simulink model "smart_irrigation_system_sim"  (R2021a)
settings: Solver=VariableStepAuto  StartTime=0.0  StopTime=10.0  RelTol=1e-3
libraries: spsBistableLib x1
settings Model: Creator=samad  LastModifiedBy=samad

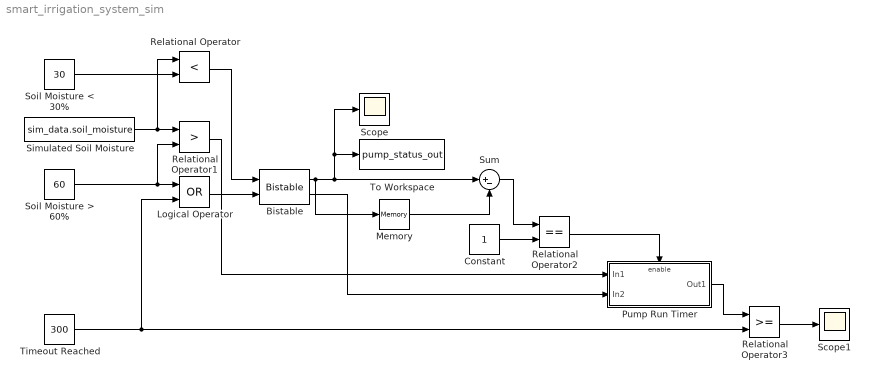
== system smart_irrigation_system_sim ==
  Bistable : spsBistableLib/Bistable  Qpriority=Set  ic=0  Ts=-1
      settings: SourceProductBaseCode=PS
  Constant : Constant
  Logical Operator : Logic  Operator=OR  AllPortsSameDT=off  OutDataTypeStr=boolean
  Memory : Memory
  Pump Run Timer : Subsystem  TreatAsAtomicUnit=on
  Relational Operator : RelationalOperator  Operator=<  OutDataTypeStr=boolean  RndMeth=Simplest
  Relational Operator1 : RelationalOperator  Operator=>  OutDataTypeStr=boolean  RndMeth=Simplest
  Relational Operator2 : RelationalOperator  Operator===  OutDataTypeStr=boolean  RndMeth=Simplest
  Relational Operator3 : RelationalOperator  OutDataTypeStr=boolean  RndMeth=Simplest
  Scope : Scope
  Scope1 : Scope
  Simulated Soil Moisture : FromWorkspace  VariableName=sim_data.soil_moisture  SampleTime=5/60
  Soil Moisture < 30% : Constant  Value=30
  Soil Moisture > 60% : Constant  Value=60
  Sum : Sum  Inputs=|+-
  Timeout Reached : Constant  Value=300
  To Workspace : ToWorkspace  VariableName=pump_status_out  SaveFormat=Timeseries  SampleTime=-1
  wires:
  Pump Run Timer/1(Out1) -> Relational Operator3/1
  Relational Operator3/1 -> Scope1/1
  Constant/1 -> Relational Operator2/2
  Bistable/1 -> To Workspace/1, Scope/1, Sum/1, Memory/1
  Soil Moisture < 30%/1 -> Relational Operator/2
  Memory/1 -> Sum/2
  Sum/1 -> Relational Operator2/1
  Logical Operator/1 -> Bistable/2
  Relational Operator1/1 -> Pump Run Timer/1(In1)
  Relational Operator/1 -> Bistable/1
  Relational Operator2/1 -> Pump Run Timer/Enable
  Simulated Soil Moisture/1 -> Relational Operator1/1, Relational Operator/1
  Soil Moisture > 60%/1 -> Relational Operator1/2, Logical Operator/1
  Timeout Reached/1 -> Logical Operator/2, Relational Operator3/2
  Bistable/2 -> Pump Run Timer/2(In2)

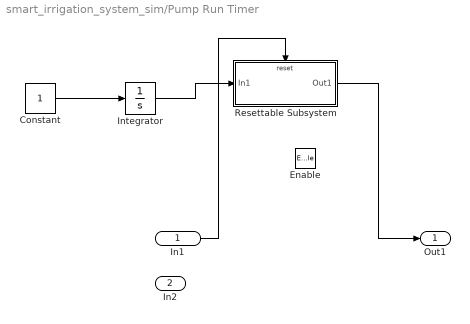
== system smart_irrigation_system_sim/Pump Run Timer ==
  In1 : Inport
  In2 : Inport  Port=2
  Enable : EnablePort
  Constant : Constant  SampleTime=10
  Integrator : Integrator
  Resettable Subsystem : Subsystem  TreatAsAtomicUnit=on
  Out1 : Outport
  wires:
  Constant/1 -> Integrator/1
  Resettable Subsystem/1(Out1) -> Out1/1
  Integrator/1 -> Resettable Subsystem/1(In1)
  In1/1 -> Resettable Subsystem/Reset

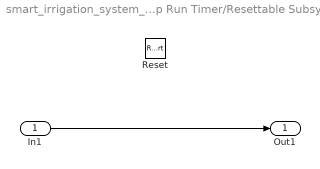
== system smart_irrigation_system_sim/Pump Run Timer/Resettable Subsystem ==
  In1 : Inport
  Reset : ResetPort  DisableCoverage=on
  Out1 : Outport
  wires:
  In1/1 -> Out1/1
